simulink model "CTRL_LO_ST1_YAWTRQSUM_test"  (R2023b)
settings: Solver=VariableStepAuto  StartTime=0.0  StopTime=10.0  RelTol=1e-3
libraries: CTRL_LO_ST1_YAWTRQSUM x1
settings Model: Creator=blatak  LastModifiedBy=blatak

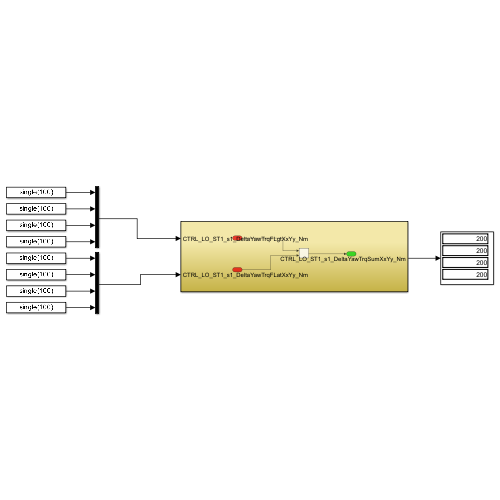
[thumbnail: Simulink's stored preview of the top-level diagram]
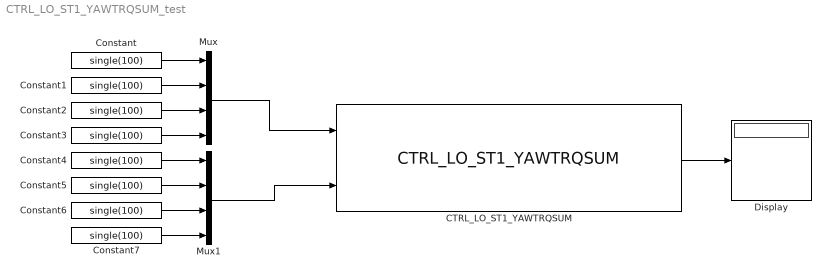
== system CTRL_LO_ST1_YAWTRQSUM_test ==
  CTRL_LO_ST1_YAWTRQSUM : CTRL_LO_ST1_YAWTRQSUM/CTRL_LO_ST1_YAWTRQSUM  SystemSampleTime=-1  VariantActivationTime=update diagram  AllowFlexibleInterface=on  Latency=0  AutoFrameSizeCalculation=off
  Constant{,1..7} (8 alike) : Constant  Value=single(100)
  Display : Display
  Mux : Mux
  Mux1 : Mux
  wires:
  Constant/1 -> Mux/1
  Constant1/1 -> Mux/2
  Constant2/1 -> Mux/3
  Constant3/1 -> Mux/4
  Constant5/1 -> Mux1/2
  Constant4/1 -> Mux1/1
  Constant7/1 -> Mux1/4
  Constant6/1 -> Mux1/3
  Mux/1 -> CTRL_LO_ST1_YAWTRQSUM/1
  Mux1/1 -> CTRL_LO_ST1_YAWTRQSUM/2
  CTRL_LO_ST1_YAWTRQSUM/1 -> Display/1
